simulink model "Lewitacja_LQR"  (R2015a)
settings: Solver=ode5  SolverMode=SingleTasking  StartTime=0.0  StopTime=1000  FixedStep=0.001  RelTol=1e-3  AbsTol=1e-6
PostLoadFcn:
  | load ML_Sensor
values from neighbouring files (symbols this model uses):
  a = a-b    (= 0.0214)    [model_nielin_zmienne.m]    (also in model_nieliniowy_zmienne.m = 0.0928)
  b = a-b    (= 0.0928)    [model_nielin_zmienne.m]    (also in model_nieliniowy_zmienne.m = 0.0214)
  g = 9.81    [model_nielin_zmienne.m]    (also in model_nieliniowy_zmienne.m)
  k = 0.2607    [model_nielin_zmienne.m]    (also in model_nieliniowy_zmienne.m)
  L = 10    [model_nielin_zmienne.m]    (also in model_nieliniowy_zmienne.m = 1)
  m = 58    [model_nielin_zmienne.m]    (also in model_nieliniowy_zmienne.m)
  T = 0.024    [model_nielin_zmienne.m]    (also in model_nieliniowy_zmienne.m)
  u_c = -0.0062    [model_nielin_zmienne.m]    (also in model_nieliniowy_zmienne.m)
  x10 = 0.010    (= 0.01)    [model_nielin_zmienne.m]    (also in model_nieliniowy_zmienne.m = 0.013)
  x20 = -1e-10    [model_nielin_zmienne.m]    (also in model_nieliniowy_zmienne.m)
  x30 = 1e-9    (= 1e-09)    [model_nielin_zmienne.m]    (also in model_nieliniowy_zmienne.m = 1e-10)
undefined symbols (not defined in the file or in its folder): K, SensorData
undefined symbols (not defined in the file): RTDAC4PCIBaseAddress
libraries: simulink x5
settings Model: SimulationMode=external  ExtModeEnableFloating=off  ExtModeTrigDuration=200000  ExtModeTrigDirection=either  ExtModeArchiveFileName=exp01.mat  ExtModeArchiveDirName=h:\temp  ExtModeWriteAllDataToWs=on  Creator=Adam Pilat  LastModifiedBy=Student
settings DataIOCC: ExternalInput=[]  InitialState=[]  LimitDataPoints=off  MaxDataPoints=5000  SignalLoggingSaveFormat=ModelDataLogs  SaveOutput=off  SaveTime=off  SignalLoggingName=sigsOut
settings OptimizationCC: BooleanDataType=off  ExpressionDepthLimit=2147483647  InitFltsAndDblsToZero=on
settings DebuggingCC: SaveWithParameterizedLinksMsg=none  UnderspecifiedInitializationDetection=Classic  MergeDetectMultiDrivingBlocksExec=none  SignalResolutionControl=TryResolveAllWithWarning  MultiTaskDSMMsg=warning  MultiTaskCondExecSysMsg=none  IntegerOverflowMsg=none  FcnCallInpInsideContextMsg=UseLocalSettings  StateNameClashWarn=warning  IntegerSaturationMsg=none
settings HardwareCC: ProdBitPerLong=64  ProdBitPerPointer=64  ProdIntDivRoundTo=Zero  ProdEndianess=LittleEndian  ProdWordSize=64  ProdHWDeviceType=Intel->x86-64  TargetBitPerLong=64  TargetBitPerPointer=64  TargetIntDivRoundTo=Zero  TargetEndianess=LittleEndian  TargetWordSize=64  TargetHWDeviceType=Intel->x86-64
settings RTWCC: SystemTargetFile=rtwin.tlc  TemplateMakefile=RTDAC_win.tmf  Description=Real-Time Windows Target
settings RTWinTargetCC: TargetFcnLib=ansi_tfl_tmw.mat  TargetPreCompLibLocation=C:\Program Files\MATLAB\R2015aSP1\toolbox\sldrt\lib\win64  ModelReferenceCompliant=off  CompOptLevelCompliant=off

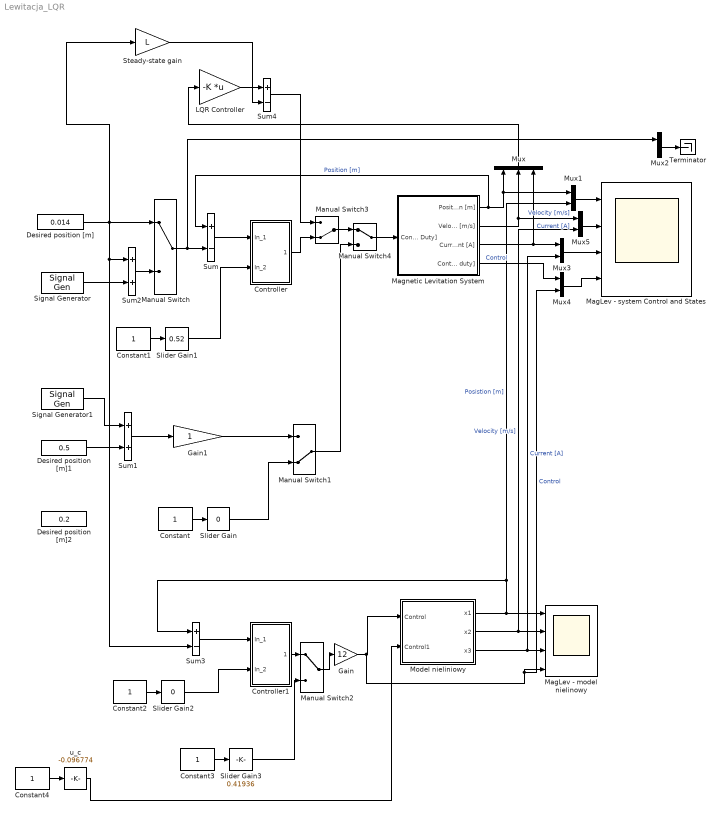
== system Lewitacja_LQR ==
  Constant{,1..4} (5 alike) : Constant
  Controller : Subsystem  mask(PID(2) Controller){P=50, I=5, D=2.5, T0=0.001}
      mask prompts: P "Proportional:"; I "Integral:"; D "Derivative:"; T0 "Sample Time:"
      mask help:
      | Enter Proportional(P), Integral(I), and Derivative(D) and divisor (N) terms.
      | P+I/s+Ds/(1/Ns+1)
      mask Help: This block implements a PID controller where parameters are entered for the Proportional, Integral and Derivative and divisor terms. Unmask this block to see how it works. The derivative term is implemented using an s/(s/N +1)  transfer function block. Making N large can create a "stiff" system.
      mask Display: disp('PID')
  Controller1 : Subsystem  mask(PID(2) Controller){P=50, I=5, D=2.5, T0=0.001}
      mask prompts: P "Proportional:"; I "Integral:"; D "Derivative:"; T0 "Sample Time:"
      mask help:
      | Enter Proportional(P), Integral(I), and Derivative(D) and divisor (N) terms.
      | P+I/s+Ds/(1/Ns+1)
      mask Help: This block implements a PID controller where parameters are entered for the Proportional, Integral and Derivative and divisor terms. Unmask this block to see how it works. The derivative term is implemented using an s/(s/N +1)  transfer function block. Making N large can create a "stiff" system.
      mask Display: disp('PID')
  Desired position [m] : Constant  Value=0.014
  Desired position [m]1 : Constant  Value=0.5
  Desired position [m]2 : Constant  Value=0.2
  Gain : Gain  Gain=12
  Gain1 : Gain
  LQR Controller : Gain  Gain=-K  Multiplication=Matrix(K*u)
  MagLev - model nielinowy : Scope  NumInputPorts=4
      settings: TimeRange=100  YMin=0.01~-0.002~-0.005~0  YMax=0.01475~0.009~0.08~0.25  SaveName=ModelNieliniowy  MaxDataPoints=10000
  MagLev - system Control and States : Scope  NumInputPorts=4
      settings: TimeRange=20  YMin=0~-100~0.25~0  YMax=2000~1000~3.5~12  SaveName=ident  MaxDataPoints=10000
  Magnetic Levitation System : Subsystem  mask(Magnetic Levitation 1 - System){BA=RTDAC4PCIBaseAddress(-1,-1), T0=0.001}
      mask prompts: BA "Base Address (dec):"; T0 "Sampling period [s]:"
      mask help:
      | MagLev1 - System connection for the real-time operating mode
      | (c) InTeCo 2005
      mask Display: image(imread('MagLev1.tif'))
  Manual Switch : ManualSwitch
  Manual Switch1 : ManualSwitch  CurrentSetting=0
  Manual Switch2 : ManualSwitch
  Manual Switch3 : ManualSwitch  CurrentSetting=0
  Manual Switch4 : ManualSwitch
  Model nieliniowy : Subsystem
  Mux : Mux  Inputs=3
  Mux{1..5} (5 alike) : Mux  Inputs=2
  Signal Generator : SignalGenerator  Amplitude=1e-3  Frequency=0.25
  Signal Generator1 : SignalGenerator  WaveForm=square  Amplitude=0.5  Frequency=200
  Slider Gain : simulink/Math Operations/Slider Gain  low=0  gain=0  high=1
  Slider Gain1 : simulink/Math Operations/Slider Gain  low=0  gain=0.52  high=1
  Slider Gain2 : simulink/Math Operations/Slider Gain  low=0  gain=0  high=1
  Slider Gain3 : simulink/Math Operations/Slider Gain  low=0  gain=0.41936  high=1
  Steady-state gain : Gain  Gain=L
  Sum : Sum  Inputs=+-  SaturateOnIntegerOverflow=on  InputSameDT=on  OutDataTypeStr=Inherit: Same as first input
  Sum1 : Sum  SaturateOnIntegerOverflow=on  InputSameDT=on  OutDataTypeStr=Inherit: Same as first input
  Sum2 : Sum  SaturateOnIntegerOverflow=on  InputSameDT=on  OutDataTypeStr=Inherit: Same as first input
  Sum3 : Sum  Inputs=+-  SaturateOnIntegerOverflow=on  InputSameDT=on  OutDataTypeStr=Inherit: Same as first input
  Sum4 : Sum  Inputs=+-  SaturateOnIntegerOverflow=on  InputSameDT=on  OutDataTypeStr=Inherit: Same as first input
  Terminator : Terminator
  u_c : simulink/Math Operations/Slider Gain  low=-1  gain=-0.096774  high=1
  wires:
  Magnetic Levitation System/1(Position [m]) -> Mux1/1, Mux/1, Sum/1  "Position [m]"
  Magnetic Levitation System/2(Velocity [m/s]) -> Mux5/1, Mux/2  "Velocity [m/s]"
  Magnetic Levitation System/3(Current [A]) -> Mux3/1, Mux/3  "Current [A]"
  Sum2/1 -> Manual Switch/2
  Signal Generator/1 -> Sum2/2
  Manual Switch/1 -> Sum/2, Mux2/1
  Sum/1 -> Controller/1(In_1)
  Mux2/1 -> Terminator/1
  Constant/1 -> Slider Gain/1
  Manual Switch4/1 -> Magnetic Levitation System/1(Control [PWM Duty])
  Desired position [m]1/1 -> Sum1/2
  Signal Generator1/1 -> Sum1/1
  Sum1/1 -> Gain1/1
  Constant1/1 -> Slider Gain1/1
  Slider Gain1/1 -> Controller/2(In_2)
  Model nieliniowy/1(x1) -> Mux1/2, Sum3/1, MagLev - model nielinowy/1  "Posistion [m]"
  Model nieliniowy/2(x2) -> Mux5/2, MagLev - model nielinowy/2  "Velocity [m/s]"
  Model nieliniowy/3(x3) -> Mux3/2, MagLev - model nielinowy/3  "Current [A]"
  Gain1/1 -> Manual Switch1/1
  Slider Gain/1 -> Manual Switch1/2
  Manual Switch1/1 -> Manual Switch4/2
  Constant2/1 -> Slider Gain2/1
  Slider Gain2/1 -> Controller1/2(In_2)
  Desired position [m]/1 -> Sum3/2, Sum2/1, Steady-state gain/1, Manual Switch/1
  Sum3/1 -> Controller1/1(In_1)
  Gain/1 -> Mux4/2, MagLev - model nielinowy/4, Model nieliniowy/1(Control)  "Control"
  Constant3/1 -> Slider Gain3/1
  Slider Gain3/1 -> Manual Switch2/2
  Controller1/1(Out_1) -> Manual Switch2/1
  Manual Switch2/1 -> Gain/1
  Mux/1 -> LQR Controller/1
  LQR Controller/1 -> Sum4/1
  Steady-state gain/1 -> Sum4/2
  Manual Switch3/1 -> Manual Switch4/1
  Controller/1(Out_1) -> Manual Switch3/2
  Sum4/1 -> Manual Switch3/1
  Mux1/1 -> MagLev - system Control and States/1
  Mux3/1 -> MagLev - system Control and States/3
  Mux4/1 -> MagLev - system Control and States/4
  Magnetic Levitation System/4(Control [PWM duty]) -> Mux4/1  "Control"
  Mux5/1 -> MagLev - system Control and States/2
  Constant4/1 -> u_c/1
  u_c/1 -> Model nieliniowy/2(Control1)

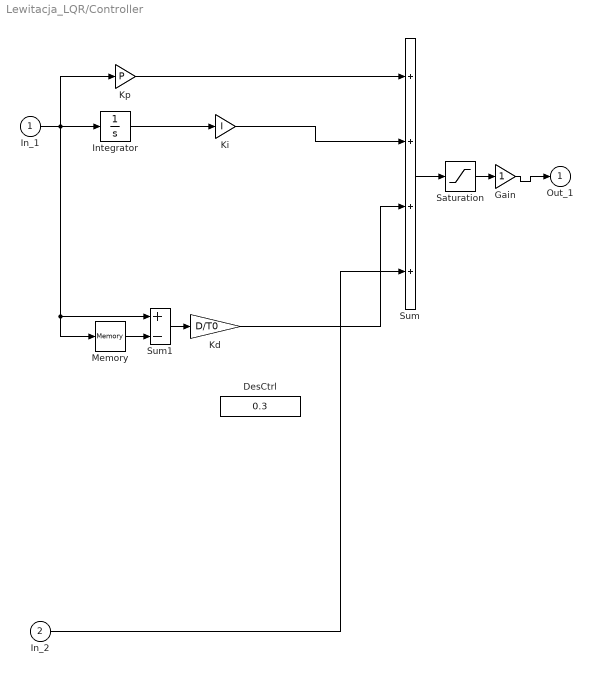
== system Lewitacja_LQR/Controller ==
  In_1 : Inport
  In_2 : Inport  Port=2
  DesCtrl : Constant  Value=0.3
  Gain : Gain  SaturateOnIntegerOverflow=on  OutDataTypeStr=Inherit: Same as input  ParamDataTypeStr=Inherit: Same as input
  Integrator : Integrator  InitialCondition=0*4e-5  LimitOutput=on  UpperSaturationLimit=1  LowerSaturationLimit=-1
  Kd : Gain  Gain=D/T0  SaturateOnIntegerOverflow=on  OutDataTypeStr=Inherit: Same as input  ParamDataTypeStr=Inherit: Same as input
  Ki : Gain  Gain=I  SaturateOnIntegerOverflow=on  OutDataTypeStr=Inherit: Same as input  ParamDataTypeStr=Inherit: Same as input
  Kp : Gain  Gain=P  SaturateOnIntegerOverflow=on  OutDataTypeStr=Inherit: Same as input  ParamDataTypeStr=Inherit: Same as input
  Memory : Memory
  Saturation : Saturate  UpperLimit=1  LowerLimit=0
  Sum : Sum  Inputs=++++  SaturateOnIntegerOverflow=on  InputSameDT=on  OutDataTypeStr=Inherit: Same as first input
  Sum1 : Sum  Inputs=+-  SaturateOnIntegerOverflow=on  InputSameDT=on  OutDataTypeStr=Inherit: Same as first input
  Out_1 : Outport  InitialOutput=0
  wires:
  Ki/1 -> Sum/2
  Integrator/1 -> Ki/1
  Sum/1 -> Saturation/1
  In_1/1 -> Kp/1, Memory/1, Sum1/1, Integrator/1
  Memory/1 -> Sum1/2
  Sum1/1 -> Kd/1
  Saturation/1 -> Gain/1
  Kp/1 -> Sum/1
  Kd/1 -> Sum/3
  Gain/1 -> Out_1/1
  In_2/1 -> Sum/4

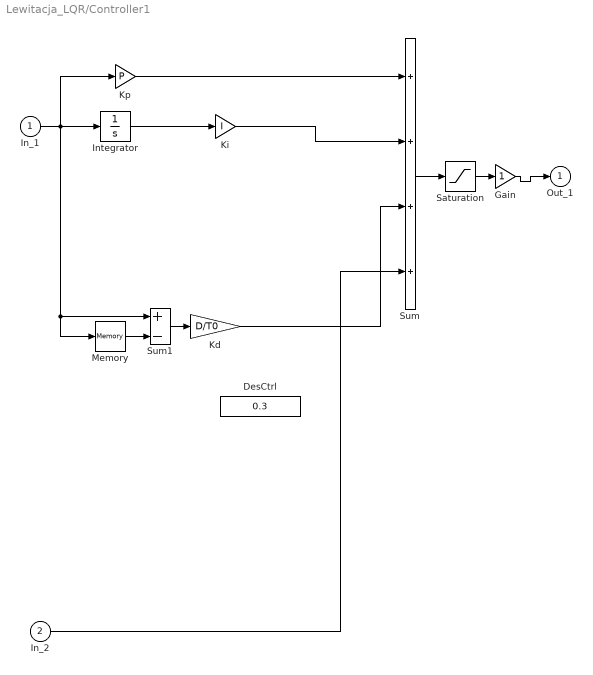
== system Lewitacja_LQR/Controller1 ==
  In_1 : Inport
  In_2 : Inport  Port=2
  DesCtrl : Constant  Value=0.3
  Gain : Gain  SaturateOnIntegerOverflow=on  OutDataTypeStr=Inherit: Same as input  ParamDataTypeStr=Inherit: Same as input
  Integrator : Integrator  InitialCondition=0*4e-5  LimitOutput=on  UpperSaturationLimit=1  LowerSaturationLimit=-1
  Kd : Gain  Gain=D/T0  SaturateOnIntegerOverflow=on  OutDataTypeStr=Inherit: Same as input  ParamDataTypeStr=Inherit: Same as input
  Ki : Gain  Gain=I  SaturateOnIntegerOverflow=on  OutDataTypeStr=Inherit: Same as input  ParamDataTypeStr=Inherit: Same as input
  Kp : Gain  Gain=P  SaturateOnIntegerOverflow=on  OutDataTypeStr=Inherit: Same as input  ParamDataTypeStr=Inherit: Same as input
  Memory : Memory
  Saturation : Saturate  UpperLimit=1  LowerLimit=0
  Sum : Sum  Inputs=++++  SaturateOnIntegerOverflow=on  InputSameDT=on  OutDataTypeStr=Inherit: Same as first input
  Sum1 : Sum  Inputs=+-  SaturateOnIntegerOverflow=on  InputSameDT=on  OutDataTypeStr=Inherit: Same as first input
  Out_1 : Outport  InitialOutput=0
  wires:
  In_2/1 -> Sum/4
  Gain/1 -> Out_1/1
  Kd/1 -> Sum/3
  Kp/1 -> Sum/1
  Saturation/1 -> Gain/1
  Sum1/1 -> Kd/1
  Memory/1 -> Sum1/2
  In_1/1 -> Integrator/1, Sum1/1, Memory/1, Kp/1
  Sum/1 -> Saturation/1
  Integrator/1 -> Ki/1
  Ki/1 -> Sum/2

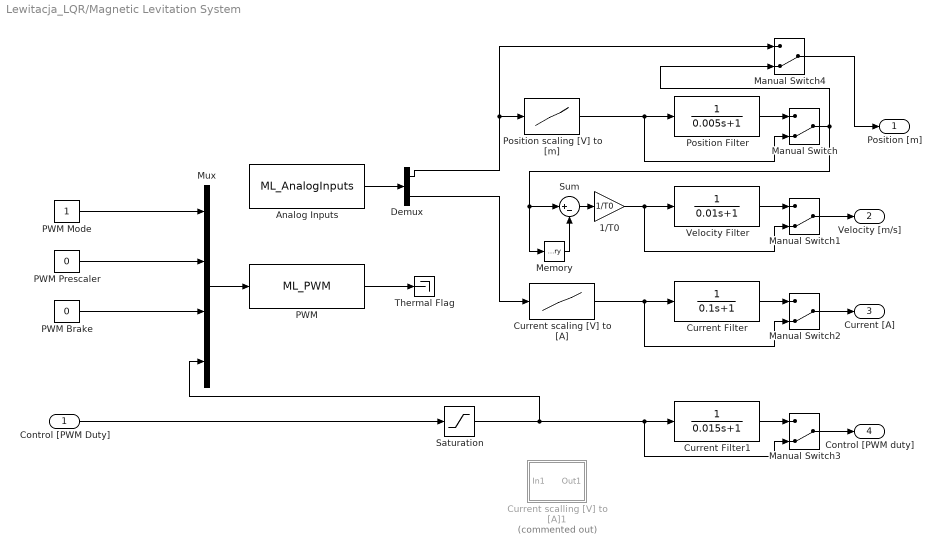
== system Lewitacja_LQR/Magnetic Levitation System ==
  Control [PWM Duty] : Inport
  1/T0 : Gain  Gain=1/T0  SaturateOnIntegerOverflow=on  OutDataTypeStr=Inherit: Same as input  ParamDataTypeStr=Inherit: Same as input
  Analog Inputs : S-Function  FunctionName=ML_AnalogInputs  Parameters=BA, [4 2], [1 1], T0
  Current Filter : TransferFcn  Denominator=[0.1 1]
  Current Filter1 : TransferFcn  Denominator=[0.015 1]
  "Current scaling [V] to [A] " : Lookup  InputValues=SensorData.Current_input  Table=SensorData.Current_output  SaturateOnIntegerOverflow=on
  Current scalling [V] to [A]1 : Subsystem  Commented=on
      mask Display: plot([0    0.5000    1.0000    1.5000    2.0000    2.5000], [-0.0317    0.4951    1.0302    1.5738    2.1258    2.6863]);
  Demux : Demux  Outputs=2
  Manual Switch{,1..4} (5 alike) : ManualSwitch  CurrentSetting=0
  Memory : Memory
  Mux : Mux
  PWM : S-Function  FunctionName=ML_PWM  Parameters=BA, T0
  PWM Brake : Constant  Value=0
  PWM Mode : Constant
  PWM Prescaler : Constant  Value=0
  Position Filter : TransferFcn  Denominator=[0.005 1]
  Position scaling [V] to [m] : Lookup  InputValues=SensorData.Sensor_V(end:-1:1)  Table=SensorData.Distance_m(end:-1:1)  SaturateOnIntegerOverflow=on
  Saturation : Saturate  UpperLimit=1  LowerLimit=0
  Sum : Sum  Inputs=|+-  SaturateOnIntegerOverflow=on  InputSameDT=on  OutDataTypeStr=Inherit: Same as first input
  Thermal Flag : Terminator
  Velocity Filter : TransferFcn  Denominator=[0.01 1]
  Position [m] : Outport
  Velocity [m/s] : Outport  Port=2
  Current [A] : Outport  Port=3
  Control [PWM duty] : Outport  Port=4
  wires:
  Current Filter/1 -> Manual Switch2/1
  Velocity Filter/1 -> Manual Switch1/1
  Manual Switch/1 -> Memory/1, Sum/1, Manual Switch4/2
  Position Filter/1 -> Manual Switch/1
  Position scaling [V] to [m]/1 -> Manual Switch/2, Position Filter/1
  "Current scaling [V] to [A] "/1 -> Manual Switch2/2, Current Filter/1
  1/T0/1 -> Manual Switch1/2, Velocity Filter/1
  Sum/1 -> 1/T0/1
  Memory/1 -> Sum/2
  Analog Inputs/1 -> Demux/1
  Mux/1 -> PWM/1
  PWM Prescaler/1 -> Mux/2
  PWM Mode/1 -> Mux/1
  PWM/1 -> Thermal Flag/1
  Saturation/1 -> Mux/4, Current Filter1/1, Manual Switch3/2
  PWM Brake/1 -> Mux/3
  Manual Switch1/1 -> Velocity [m/s]/1
  Control [PWM Duty]/1 -> Saturation/1
  Current Filter1/1 -> Manual Switch3/1
  Demux/1 -> Manual Switch4/1, Position scaling [V] to [m]/1
  Manual Switch4/1 -> Position [m]/1
  Demux/2 -> "Current scaling [V] to [A] "/1
  Manual Switch2/1 -> Current [A]/1
  Manual Switch3/1 -> Control [PWM duty]/1

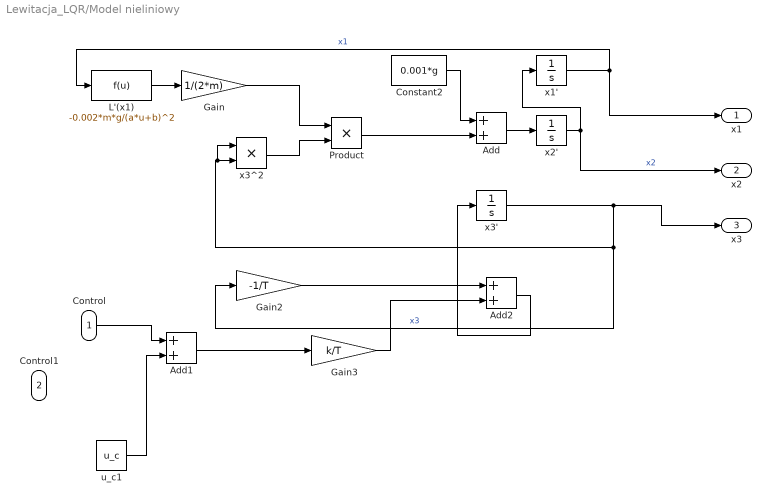
== system Lewitacja_LQR/Model nieliniowy ==
  Control : Inport
  Control1 : Inport  Port=2
  Add : Sum
  Add1 : Sum
  Add2 : Sum
  Constant2 : Constant  Value=0.001*g
  Gain : Gain  Gain=1/(2*m)
  Gain2 : Gain  Gain=-1/T
  Gain3 : Gain  Gain=k/T
  L'(x1) : Fcn  Expr=-0.002*m*g/(a*u+b)^2
  Product : Product
  u_c1 : Constant  Value=u_c
  x1' : Integrator  InitialCondition=x10  UpperSaturationLimit=0.02  LowerSaturationLimit=0
  x2' : Integrator  InitialCondition=x20
  x3' : Integrator  InitialCondition=x30
  x3^2 : Product
  x1 : Outport
  x2 : Outport  Port=2
  x3 : Outport  Port=3
  wires:
  Control/1 -> Add1/1
  x1'/1 -> x1/1, L'(x1)/1  "x1"
  L'(x1)/1 -> Gain/1
  Gain/1 -> Product/1
  x3^2/1 -> Product/2
  x2'/1 -> x2/1, x1'/1  "x2"
  Add/1 -> x2'/1
  Constant2/1 -> Add/1
  Product/1 -> Add/2
  Add2/1 -> x3'/1
  Gain2/1 -> Add2/1
  Gain3/1 -> Add2/2
  Add1/1 -> Gain3/1
  x3'/1 -> Gain2/1, x3^2/1, x3^2/2, x3/1  "x3"
  u_c1/1 -> Add1/2

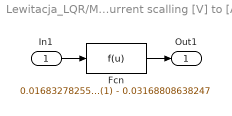
== system Lewitacja_LQR/Magnetic Levitation System/Current scalling [V] to [A]1 ==
  In1 : Inport
  Fcn : Fcn  Expr=0.01683278255001*u(1)^2 +1.04509985660788*u(1) - 0.03168808638247
  Out1 : Outport
  wires:
  Fcn/1 -> Out1/1
  In1/1 -> Fcn/1
